simulink model "NewWatch"  (R2017a)
settings: Solver=ode3  StartTime=0.0  StopTime=inf  FixedStep=0.1  RelTol=1e-3
libraries: simulink x1
settings Model: Creator=admim  LastModifiedBy=gabrieleserra
settings DataIOCC: LimitDataPoints=on  SaveFormat=Structure
settings OptimizationCC: DefaultParameterBehavior=Inlined  InlineInvariantSignals=on  LifeSpan=Inf
settings DebuggingCC: SolverPrmCheckMsg=warning  AllowSymbolicDim=off  SFUnexpectedBacktrackingDiag=warning  SFNoUnconditionalDefaultTransitionDiag=warning  SFExecutionAtInitializationDiag=none
settings HardwareCC: ProdBitPerPointer=32  ProdBitPerSizeT=32  ProdBitPerPtrDiffT=32  ProdLargestAtomicFloat=None  ProdIntDivRoundTo=Undefined  ProdEndianess=Unspecified  ProdWordSize=32  ProdHWDeviceType=32-bit Generic
settings ModelReferenceCC: PropagateSignalLabelsOutOfModel=off
settings SFSimCC: MATLABDynamicMemAlloc=off
settings RTWCC: SystemTargetFile=ert.tlc  GenCodeOnly=on  TemplateMakefile=ert_default_tmf  Description=Embedded Coder
settings CodeAppCC: IgnoreCustomStorageClasses=off
settings ERTTargetCC: MultiwordLength=2048  IncludeMdlTerminateFcn=off  SuppressErrorStatus=on  SupportAbsoluteTime=off  MultiInstanceERTCode=on  CodeInterfacePackaging=Reusable function  SupportNonFinite=off  SupportComplex=off  PurelyIntegerCode=on  InlinedParameterPlacement=NonHierarchical  MultiInstanceErrorCode=None  ERTCustomFileTemplate=example_file_process.tlc  ConvertIfToSwitch=off  SuppressUnreachableDefaultCases=off
settings ConfigComp: CovMetricSettings=dw  CovHtmlReporting=on  CovSaveCumulativeToWorkspaceVar=on  CovSaveSingleToWorkspaceVar=on  CovExternalEMLEnable=off  CovSFcnEnable=off

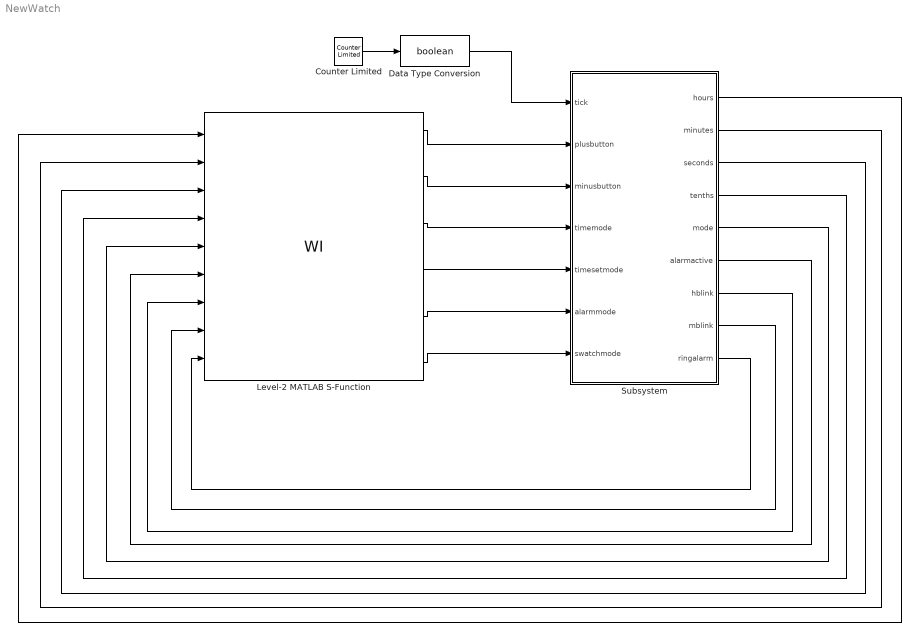
== system NewWatch ==
  Counter Limited : simulink/Sources/Counter Limited  uplimit=1  tsamp=0.1
  Data Type Conversion : DataTypeConversion  OutDataTypeStr=boolean
  Level-2 MATLAB S-Function : M-S-Function  FunctionName=WI
      mask Display:
      | port_label('input', 1, 'hours')
      | port_label('input', 2, 'minutes')
      | port_label('input', 3, 'seconds')
      | port_label('input', 4, 'tenths')
      | port_label('input', 5, 'mode')
      | port_label('input', 6, 'alarmactive')
      | port_label('input', 7, 'hblink')
      | port_label('input', 8, 'mblink')
      | port_label('input', 9, 'ringalarm')
      | 
      | port_label('output', 1, 'plus')
      | port_label('output', 2, 'minus')
      | port_label('output', 3, 'time')
      | port_label('output', 4, 'time set')
      | port_label('output', 5, 'alarm')
      | port_label('output', 6, 'stopwatch')
  Subsystem : Subsystem
  wires:
  Counter Limited/1 -> Data Type Conversion/1
  Data Type Conversion/1 -> Subsystem/1(tick)
  Level-2 MATLAB S-Function/1 -> Subsystem/2(plusbutton)
  Level-2 MATLAB S-Function/2 -> Subsystem/3(minusbutton)
  Level-2 MATLAB S-Function/3 -> Subsystem/4(timemode)
  Level-2 MATLAB S-Function/4 -> Subsystem/5(timesetmode)
  Level-2 MATLAB S-Function/5 -> Subsystem/6(alarmmode)
  Level-2 MATLAB S-Function/6 -> Subsystem/7(swatchmode)
  Subsystem/1(hours) -> Level-2 MATLAB S-Function/1
  Subsystem/2(minutes) -> Level-2 MATLAB S-Function/2
  Subsystem/3(seconds) -> Level-2 MATLAB S-Function/3
  Subsystem/4(tenths) -> Level-2 MATLAB S-Function/4
  Subsystem/5(mode) -> Level-2 MATLAB S-Function/5
  Subsystem/7(hblink) -> Level-2 MATLAB S-Function/7
  Subsystem/8(mblink) -> Level-2 MATLAB S-Function/8
  Subsystem/6(alarmactive) -> Level-2 MATLAB S-Function/6
  Subsystem/9(ringalarm) -> Level-2 MATLAB S-Function/9

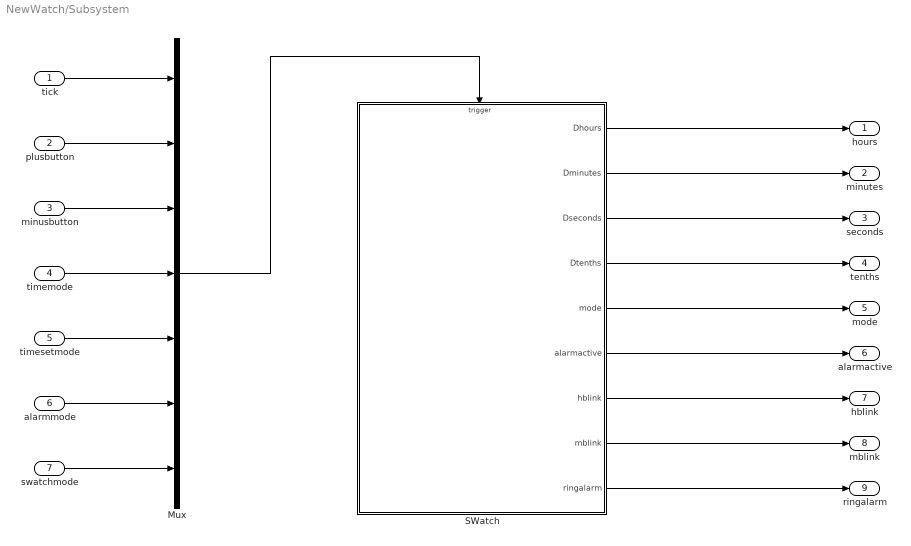
== system NewWatch/Subsystem ==
  tick : Inport
  plusbutton : Inport  Port=2
  minusbutton : Inport  Port=3
  timemode : Inport  Port=4
  timesetmode : Inport  Port=5
  alarmmode : Inport  Port=6
  swatchmode : Inport  Port=7
  Mux : Mux  Inputs=7
  SWatch : Stateflow chart  TreatAsAtomicUnit=on
  hours : Outport
  minutes : Outport  Port=2
  seconds : Outport  Port=3
  tenths : Outport  Port=4
  mode : Outport  Port=5
  alarmactive : Outport  Port=6
  hblink : Outport  Port=7
  mblink : Outport  Port=8
  ringalarm : Outport  Port=9
  wires:
  SWatch/4(Dtenths) -> tenths/1
  SWatch/3(Dseconds) -> seconds/1
  SWatch/5(mode) -> mode/1
  swatchmode/1 -> Mux/7
  alarmmode/1 -> Mux/6
  timesetmode/1 -> Mux/5
  timemode/1 -> Mux/4
  minusbutton/1 -> Mux/3
  plusbutton/1 -> Mux/2
  Mux/1 -> SWatch/Trigger
  tick/1 -> Mux/1
  SWatch/2(Dminutes) -> minutes/1
  SWatch/7(hblink) -> hblink/1
  SWatch/8(mblink) -> mblink/1
  SWatch/9(ringalarm) -> ringalarm/1
  SWatch/1(Dhours) -> hours/1
  SWatch/6(alarmactive) -> alarmactive/1

== stateflow chart NewWatch/Subsystem/SWatch ==
  settings: executeAtInitialization=1
  state ControlSystem [parallel]
    settings: executionOrder=1
    state timesetmode
      en:mode=uint8(1); hblink=false; mblink=false;counth=uint8(0);countm=uint8(0);
      ex:hblink=false; mblink=false;counth=uint8(0);countm=uint8(0);
      note: % entry in timesetmod: set mode to 1 and reset vars
          | % exit from timesetmod: reset blink vars
      note: % if minute is 0, re-start from 59
      note: % if hour is 0, re-start from 23
      note: % subtract 1 hour
      note: % subtract 1 minute
      state sethours
        en: Dhours = hours;
        note: % (re)entry in sethour state:
            | % update current hour digit
      state setminutes
        en: Dminutes = minutes;hblink=false;
        note: % (re)entry in setminutes state:
            | % update current minute digit
      note: % every 5 tick, enable/disable blink
      note: % display on screen current timestamp
      note: % switch from hour-set to minute-set
          | % and vice versa, updating the blink var
      note: % each tick increment countm var
      note: % add 1 hour
      note: % every 5 tick, enable/disable blink
      note: % add 1 minute
      note: % each tick increment counth var
      sethours -> sethours [order 2] : Bminus[hours == 0]/{hours = uint8(23)}
      sethours -> sethours [order 3] : Bminus/{hours = hours -1}
      setminutes -> setminutes [order 2] : Bminus[minutes == 0]/{minutes = uint8(59)}
      setminutes -> setminutes [order 3] : Bminus/{minutes = minutes -1}
      sethours -> setminutes [order 4] : Btimeset/{counth=uint8(0);hblink=false}
      (junction 242) -> setminutes [order 1] : ttick[countm == 0]/{mblink = ~mblink}
      (default) -> sethours : {Dhours=hours;Dminutes=minutes}
      setminutes -> (junction 242) [order 5] : ttick/{countm = mod (countm + 1,5)}
      (junction 242) -> setminutes [order 2]
      setminutes -> sethours [order 4] : Btimeset/{countm=uint8(0);mblink=false}
      sethours -> sethours [order 1] : Bplus/{hours = mod(hours+1,24)}
      (junction 239) -> sethours [order 2]
      sethours -> (junction 239) [order 5] : ttick/{counth = mod (counth + 1,5)}
      (junction 239) -> sethours [order 1] : ttick[counth == 0]/{hblink = ~hblink}
      setminutes -> setminutes [order 1] : Bplus/{minutes = mod(minutes+1,60)}
    state timemode
      en:mode=uint8(0);
      du: Dhours=hours;Dminutes=minutes;Dseconds=seconds;
      note: % entry in timemode state: mode is set to 0
          | % during timemode state: update displayed digits
    state stopwatchmode
      en:mode=uint8(3);
      note: % entry in stopwatch state: mode is set to 3
      note: % stopwatch variables are reset when stopwatch mode is selected
      state stopped
        en: Dhours = SWhours; Dminutes = SWminutes; Dseconds = SWseconds; Dtenths = SWtenths; SWlap = false;
        note: % entry in stopped state: refresh displayed digits, avoiding other modes digits in display
      state running
        note: % another second is passed away
            | % reset tenths and add 1 second
        note: % another minute is passed away
            | % reset seconds and add 1 minute
        note: % increment the number of tenths every tick
        note: % another hour is passed away
            | % reset minute and add 1 hour
        note: % if lap mode is disabled, refresh displayed digits
        state counting
        (junction 97) -> (junction 99) [order 1] : [SWtenths==0]{SWseconds=mod(SWseconds+1, 60)}
        (junction 99) -> (junction 94) [order 1] : [SWseconds==0]{SWminutes=mod(SWminutes+1, 60)}
        (junction 94) -> (junction 96) [order 2]
        (junction 97) -> (junction 96) [order 2]
        (junction 94) -> (junction 96) [order 1] : [SWminutes==0]{SWhours=mod(SWhours+1,24)}
        (junction 99) -> (junction 96) [order 2]
        counting -> (junction 97) : ttick {SWtenths=mod(SWtenths+1,10)}
        (junction 96) -> counting [order 2]
        (junction 96) -> counting [order 1] : [SWlap==false]{Dhours = SWhours; Dminutes = SWminutes; Dseconds = SWseconds; Dtenths = SWtenths;}
        (default) -> counting
      note: % when running, if Bminus is pressed, lap mode is enabled/disabled
      (default) -> stopped : {SWhours = uint8(0); SWminutes = uint8(0); SWseconds = uint8(0); SWtenths = uint8(0); SWlap = false;}
      stopped -> running : Bplus
      running -> stopped [order 1] : Bplus
      running -> running [order 2] : Bminus{SWlap = not(SWlap)}
    state alarmmode
      en:mode=uint8(2); hblink=false;mblink=false;counth=uint8(0);countm=uint8(0); alarmactive=false;
      ex:hblink=false;mblink=false;counth=uint8(0);countm=uint8(0);
      note: % entry in timesetmod: set mode to 2 and reset vars
          | % exit from timesetmod: reset blink vars
      note: % if hour is 0, re-start from 23
      note: % subtract 1 hour
      note: % if minute is 0, re-start from 59
      note: % subtract 1 minute
      state setAhours
        en: Dhours = Ahours;
        note: % (re)entry in setAhour state:
            | % update current hour digit
      state setAminutes
        en: Dminutes = Aminutes;
        note: % (re)entry in setAminutes state:
            | % update current minute digit
      note: % every 5 tick, enable/disable blink
      note: % switch from alarm hour-set to alarm
          | % minute-set and vice versa
          | % updating the blink var
      note: % display on screen current timestamp
      note: % return in set mode
      note: % each tick increment countm var
      note: % every 5 tick, enable/disable blink
      note: % add 1 minute
      note: % add 1 hour
      note: % with the third tap stop blinking and activate alarm
      note: % each tick increment counth var
      state switchOnAlarm
        en: alarmactive=true;
      setAhours -> setAhours [order 2] : Bminus[Ahours == 0]/{Ahours = uint8(23)}
      setAhours -> setAhours [order 3] : Bminus/{Ahours = Ahours -1}
      setAminutes -> setAminutes [order 2] : Bminus[Aminutes == 0]/{Aminutes = uint8(59)}
      setAminutes -> setAminutes [order 3] : Bminus/{Aminutes =Aminutes -1}
      setAhours -> setAminutes [order 4] : Balarm/{counth=uint8(0);hblink=false}
      (junction 246) -> setAminutes [order 1] : ttick[countm ==0]/{mblink = ~mblink}
      (default) -> setAhours : {Dhours = Ahours; Dminutes = Aminutes}
      setAminutes -> (junction 246) [order 5] : ttick/{countm = mod (countm+ 1,5)}
      (junction 246) -> setAminutes [order 2]
      switchOnAlarm -> setAhours : Balarm{alarmactive=false;}
      setAminutes -> switchOnAlarm [order 4] : Balarm/{countm=uint8(0);mblink=false}
      setAminutes -> setAminutes [order 1] : Bplus/{Aminutes = mod(Aminutes+1,60)}
      setAhours -> setAhours [order 1] : Bplus/{Ahours = mod(Ahours+1,24)}
      (junction 234) -> setAhours [order 1] : ttick[counth == 0]/{hblink = ~hblink}
      setAhours -> (junction 234) [order 5] : ttick/{counth = mod (counth + 1,5)}
      (junction 234) -> setAhours [order 2]
    (default) -> timemode
    timesetmode -> timemode [order 2] : Btime
    timemode -> timesetmode [order 1] : Btimeset
    timemode -> stopwatchmode [order 2] : Bstop
    stopwatchmode -> timemode [order 2] : Btime
    alarmmode -> timemode [order 3] : Btime
    timemode -> alarmmode [order 3] : Balarm
    timesetmode -> stopwatchmode [order 1] : Bstop
    stopwatchmode -> timesetmode [order 1] : Btimeset
    alarmmode -> timesetmode [order 1] : Btimeset
    timesetmode -> alarmmode [order 3] : Balarm
    stopwatchmode -> alarmmode [order 3] : Balarm
    alarmmode -> stopwatchmode [order 2] : Bstop
  state TimeCount [parallel]
    settings: executionOrder=2
    note: % reset time when Stopwatch is switch ON
    note: % increment the number of tenths every tick
    state timecount
    note: % another second is passed away
        | % reset tenths and add 1 second
    note: % another minute is passed away
        | % reset seconds and add 1 minute
    note: % another hour is passed away
        | % reset minute and add 1 hour
    (default) -> timecount : /{hours=uint8(0);minutes=uint8(0);seconds=uint8(0);tenths=uint8(0)}
    timecount -> (junction 20) : ttick {tenths=mod(tenths+1,10)}
    (junction 20) -> (junction 34) [order 2]
    (junction 20) -> (junction 28) [order 1] : [tenths==0]{seconds=mod(seconds+1, 60)}
    (junction 28) -> (junction 34) [order 2]
    (junction 34) -> timecount
    (junction 28) -> (junction 31) [order 1] : [seconds==0]{minutes=mod(minutes+1, 60)}
    (junction 31) -> (junction 34) [order 2]
    (junction 31) -> timecount [order 1] : [minutes==0]{hours=mod(hours+1,24)}
  state AlarmManage [parallel]
    en: alarmactive=false;ringalarm=false;countalarm=uint8(0);
    settings: executionOrder=3
    note: % entry in AlarmManage state: reset alarm vars
    note: % if alarm is active and timestamp is the chosen one
        | % go from silent to ringing
    state ringing
    state silent
    note: % reset alarm hour and minute
    note: % if alarm is disable or timestap is no more the chosen one
        | % return from ringing to silent and disable alarm
    note: % every 5 tick, enable/disable blink
    note: % each tick increment counth var
    silent -> ringing : [hours == Ahours && minutes == Aminutes && alarmactive == true ]
    (default) -> silent : {Ahours = uint8(0); Aminutes = uint8(0)}
    ringing -> silent [order 1] : [ Ahours ~= hours || Aminutes ~= minutes || alarmactive == false]/{ringalarm=false}
    (junction 250) -> ringing [order 1] : ttick[countalarm== 0]/{ringalarm = ~ringalarm}
    ringing -> (junction 250) [order 2] : ttick/{countalarm=mod(countalarm+1,5)}
    (junction 250) -> ringing [order 2]
  data: hours local uint8; minutes local uint8; seconds local uint8; tenths local uint8; Dhours output uint8; Dminutes output uint8; Dseconds output uint8; Dtenths output uint8; mode output uint8; alarmactive output boolean; SWhours local uint8; SWminutes local uint8; SWseconds local uint8; SWtenths local uint8; Ahours local uint8 =uint8(0); Aminutes local uint8 =uint8(0); hblink output boolean; mblink output boolean; ringalarm output boolean; counth local uint8 =uint8(0); countm local uint8 =uint8(0); countalarm local uint8 =uint8(0); SWlap local boolean =false
  events: ttick input EITHER_EDGE_EVENT; Bplus input RISING_EDGE_EVENT; Bminus input RISING_EDGE_EVENT; Btime input RISING_EDGE_EVENT; Btimeset input RISING_EDGE_EVENT; Balarm input RISING_EDGE_EVENT; Bstop input RISING_EDGE_EVENT
